simulink model "Simulink_4DOF_Model"  (R2023a)
settings: Solver=VariableStepAuto  StartTime=0.0  StopTime=10.0  RelTol=1e-3
InitFcn:
  | data = readtable("car_rig_data.xlsx");
settings Model: Creator=Sebastian  LastModifiedBy=Sebastian

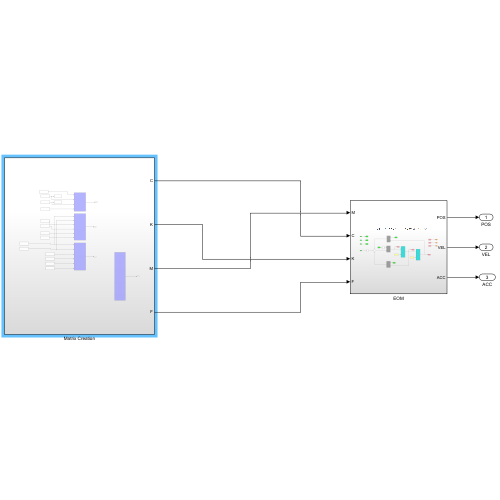
[thumbnail: Simulink's stored preview of the top-level diagram]
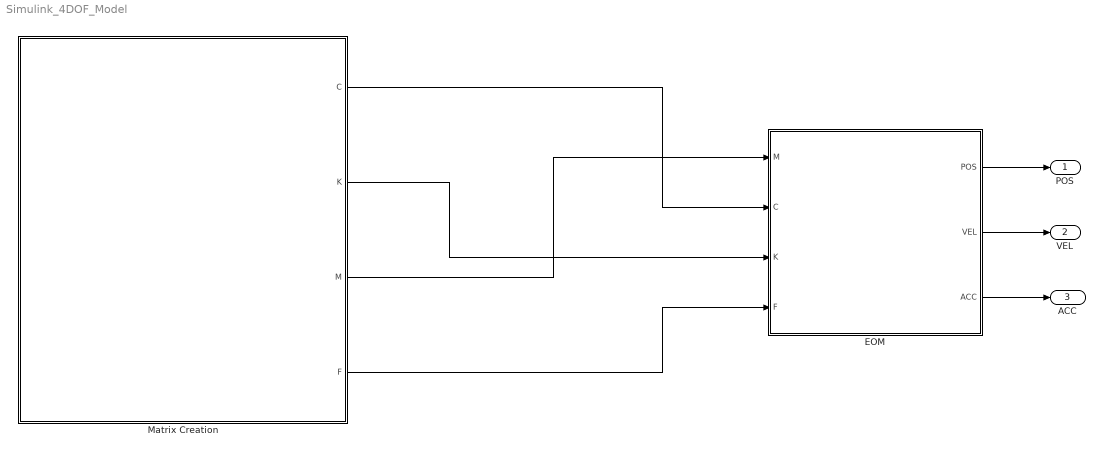
== system Simulink_4DOF_Model ==
  EOM : Subsystem
  Matrix Creation : Subsystem
  POS : Outport
  VEL : Outport  Port=2
  ACC : Outport  Port=3
  wires:
  Matrix Creation/3(M) -> EOM/1(M)
  Matrix Creation/2(K) -> EOM/3(K)
  Matrix Creation/1(C) -> EOM/2(C)
  Matrix Creation/4(F) -> EOM/4(F)
  EOM/1(POS) -> POS/1
  EOM/2(VEL) -> VEL/1
  EOM/3(ACC) -> ACC/1

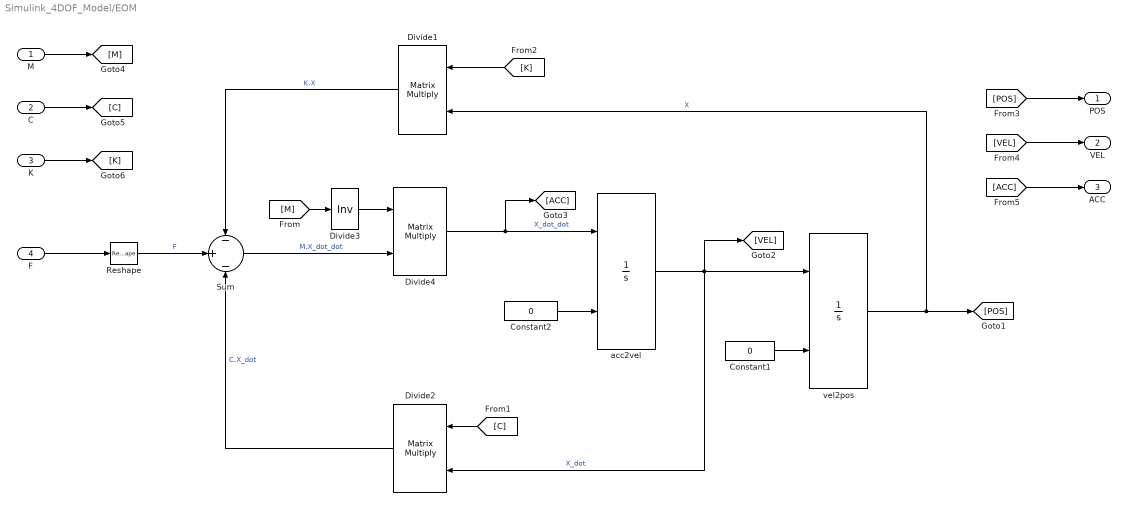
== system Simulink_4DOF_Model/EOM ==
  M : Inport
  C : Inport  Port=2
  K : Inport  Port=3
  F : Inport  Port=4
  Constant1 : Constant  Value=0  VectorParams1D=off
  Constant2 : Constant  Value=0  VectorParams1D=off
  Divide1 : Product  Multiplication=Matrix(*)
  Divide2 : Product  Multiplication=Matrix(*)
  Divide3 : Product  Inputs=/  Multiplication=Matrix(*)
  Divide4 : Product  Multiplication=Matrix(*)
  Reshape : Reshape  OutputDimensionality=Column vector (2-D)
  Sum : Sum  Inputs=-|+|-
  acc2vel : Integrator  InitialConditionSource=external
  vel2pos : Integrator  InitialConditionSource=external
  POS : Outport
  VEL : Outport  Port=2
  ACC : Outport  Port=3
  wires:
  Divide4/1 -> [ACC], acc2vel/1  "X_dot_dot"
  [C] -> Divide2/1
  vel2pos/1 -> [POS], Divide1/2  "X"
  Divide1/1 -> Sum/1  "K.X"
  acc2vel/1 -> vel2pos/1, [VEL], Divide2/2  "X_dot"
  [K] -> Divide1/1
  C/1 -> [C]
  Constant2/1 -> acc2vel/2
  F/1 -> Reshape/1
  [ACC] -> ACC/1
  [M] -> Divide3/1
  Constant1/1 -> vel2pos/2
  [VEL] -> VEL/1
  Sum/1 -> Divide4/2  "M.X_dot_dot"
  Divide2/1 -> Sum/3  "C.X_dot"
  Divide3/1 -> Divide4/1
  Reshape/1 -> Sum/2  "F"
  [POS] -> POS/1
  M/1 -> [M]
  K/1 -> [K]

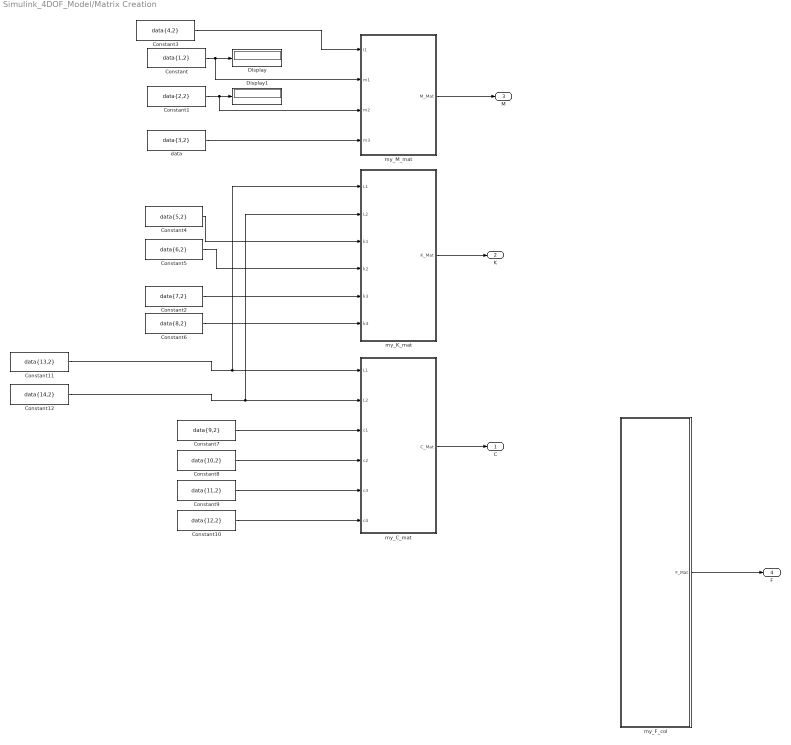
== system Simulink_4DOF_Model/Matrix Creation ==
  Constant : Constant  Value=data{1,2}
  Constant1 : Constant  Value=data{2,2}
  Constant10 : Constant  Value=data{12,2}
  Constant11 : Constant  Value=data{13,2}
  Constant12 : Constant  Value=data{14,2}
  Constant2 : Constant  Value=data{7,2}
  Constant3 : Constant  Value=data{4,2}
  Constant4 : Constant  Value=data{5,2}
  Constant5 : Constant  Value=data{6,2}
  Constant6 : Constant  Value=data{8,2}
  Constant7 : Constant  Value=data{9,2}
  Constant8 : Constant  Value=data{10,2}
  Constant9 : Constant  Value=data{11,2}
  Display : Display
  Display1 : Display
  data : Constant  Value=data{3,2}
  my_C_mat : MATLAB Function  TreatAsAtomicUnit=on
  my_F_col : MATLAB Function  TreatAsAtomicUnit=on
  my_K_mat : MATLAB Function  TreatAsAtomicUnit=on
  my_M_mat : MATLAB Function  TreatAsAtomicUnit=on
  C : Outport
  K : Outport  Port=2
  M : Outport  Port=3
  F : Outport  Port=4
  wires:
  my_F_col/1(F_Mat) -> F/1
  my_C_mat/1(C_Mat) -> C/1
  my_K_mat/1(K_Mat) -> K/1
  my_M_mat/1(M_Mat) -> M/1
  Constant/1 -> my_M_mat/2(m1), Display/1
  Constant1/1 -> my_M_mat/3(m2), Display1/1
  Constant3/1 -> my_M_mat/1(I1)
  data/1 -> my_M_mat/4(m3)
  Constant5/1 -> my_K_mat/4(k2)
  Constant4/1 -> my_K_mat/3(k1)
  Constant2/1 -> my_K_mat/5(k3)
  Constant6/1 -> my_K_mat/6(k4)
  Constant10/1 -> my_C_mat/6(c4)
  Constant9/1 -> my_C_mat/5(c3)
  Constant8/1 -> my_C_mat/4(c2)
  Constant7/1 -> my_C_mat/3(c1)
  Constant11/1 -> my_K_mat/1(L1), my_C_mat/1(L1)
  Constant12/1 -> my_C_mat/2(L2), my_K_mat/2(L2)

== matlab function Simulink_4DOF_Model/Matrix Creation/my_C_mat ==
  data: L1 input; C_Mat output; L2 input; c1 input; c2 input; c3 input; c4 input
function C_Mat = my_C_mat(L1,L2,c1,c2,c3,c4)
%#codegen

%    This function was generated by the Symbolic Math Toolbox version 9.3.
%    29-May-2023 20:31:21

% L1 = complex(L1);  % if required to enforce complex operations
% L2 = complex(L2);  % if required to enforce complex operations
% c1 = complex(c1);  % if required to enforce complex operations
% c2 = complex(c2);  % if required to enforce complex operations
% c3 = complex(c3);  % if required to enforce complex operations
% c4 = complex(c4);  % if required to enforce complex operations
t2 = L1.*c1;
t3 = L2.*c2;
t4 = -c1;
t5 = -c2;
C_Mat = reshape([t4+t5,-t2+t3,t4,t5,t2+t3,L1.*t2-L2.*t3,t2,t3,c1,t2,c1+c3,0.0,c2,-t3,0.0,c2+c4],[4,4]);
end

== matlab function Simulink_4DOF_Model/Matrix Creation/my_M_mat ==
  data: I1 input; M_Mat output; m1 input; m2 input; m3 input
function M_Mat = my_M_mat(I1,m1,m2,m3)
%#codegen

%    This function was generated by the Symbolic Math Toolbox version 9.3.
%    29-May-2023 20:31:20

% I1 = complex(I1);  % if required to enforce complex operations
% m1 = complex(m1);  % if required to enforce complex operations
% m2 = complex(m2);  % if required to enforce complex operations
% m3 = complex(m3);  % if required to enforce complex operations
M_Mat = reshape([m1,0.0,0.0,0.0,0.0,I1,0.0,0.0,0.0,0.0,m2,0.0,0.0,0.0,0.0,m3],[4,4]);
end

== matlab function Simulink_4DOF_Model/Matrix Creation/my_K_mat ==
  data: L1 input; K_Mat output; L2 input; k1 input; k2 input; k3 input; k4 input
function K_Mat = my_K_mat(L1,L2,k1,k2,k3,k4)
%#codegen

%    This function was generated by the Symbolic Math Toolbox version 9.3.
%    29-May-2023 20:31:21

% L1 = complex(L1);  % if required to enforce complex operations
% L2 = complex(L2);  % if required to enforce complex operations
% k1 = complex(k1);  % if required to enforce complex operations
% k2 = complex(k2);  % if required to enforce complex operations
% k3 = complex(k3);  % if required to enforce complex operations
% k4 = complex(k4);  % if required to enforce complex operations
t2 = L1.*k1;
t3 = L2.*k2;
t4 = -k1;
t5 = -k2;
K_Mat = reshape([t4+t5,-t2+t3,t4,t5,t2+t3,L1.*t2-L2.*t3,t2,t3,k1,t2,k1+k3,0.0,k2,-t3,0.0,k2+k4],[4,4]);
end

== matlab function Simulink_4DOF_Model/Matrix Creation/my_F_col ==
  data: F_Mat output
function F_Mat = my_F_col
%#codegen

%    This function was generated by the Symbolic Math Toolbox version 9.3.
%    29-May-2023 20:31:22

F_Mat = [0.0;0.0;0.0;0.0];
end
